simulink model "PubIfDecisionTOS_MDL"  (R2020b)
settings: configuration reference "DspaceConfig" (kept outside this file)
PostLoadFcn:
  | if any(exist('dsrtsu_mdlpostloadfcn', 'file') ~= 0), dsrtsu_mdlpostloadfcn('Execute', bdroot); end
InitFcn:
  | , if any(exist('dsmpb_private', 'file') ~= 0), dsmpb_private('dsmpb_mdlclblib', 'Init', bdroot); end,
undefined symbols (not defined in the file or in its folder): C_TOS_ACCEgoRAxletoFbumplength_m, C_TOS_ACCTargetFront_Flag, C_TOS_AEBJAPedObjDxThre_Val, C_TOS_AEBJAPedObjDyThre_Val, C_TOS_AEBJATargetSize_Val, C_TOS_AEBJAVehObjDxThre_Val, C_TOS_AEBJAVehObjDyThre_Val, C_TOS_AEBJuncPedTargetSize_Val, C_TOS_AEBLatObjDxThre_Val, C_TOS_AEBLatPedDyThre_Val, C_TOS_AEBLatTargetSize_Val, C_TOS_AEBLongTargetInEgoFront_Flag, C_TOS_axAbsGround_Parameter, C_TOS_CameraConfirmedFlag, C_TOS_CNsubjWidth, C_TOS_CurrentLaneCoreMinWidth_Val, C_TOS_CutInProb_Val_Zero, C_TOS_CutOutProb_Val_Zero, C_TOS_D2R_Val, C_TOS_DefaultValueObjectToCenterLine_dy, C_TOS_EgoCarWidth_Val, C_TOS_EgoDxRefPoint_m, C_TOS_EgoRAxletoFbumplength_m, C_TOS_HalfWidthVehicle_Con, C_TOS_HWA_CurrentLaneFlag, C_TOS_HWA_LeftLaneFlag, C_TOS_HWA_MovingDir_Vaild, C_TOS_HWA_MovState_Vaild, C_TOS_HWA_RightLaneFlag, C_TOS_LaneLineCourseErrorFront, C_TOS_LaneLineCourseErrorRear, C_TOS_MotorbikeDefaultWidth_m, C_TOS_NumberOfEffectiveTargets, C_TOS_Obj_Age_Val, C_TOS_Objdx_Constraint_Val, C_TOS_ObjectDefaultWidth_m, C_TOS_ObjInCurrentLane_Val, C_TOS_ObjInCurrentLaneValid, C_TOS_ObjInLeftLaneValid, C_TOS_ObjInRightLaneValid, C_TOS_ObjNotInCurrentLane_Val, C_TOS_ObjNotREElementType, C_TOS_ObjPredictDis_dy_ConstantVal_Zeros, C_TOS_ObjToCenterLine_ConstantVal_Zeros, C_TOS_OFMObjIDInvilad_Val, C_TOS_PIL_LatDisCons_Val_zero, C_TOS_PIL_ObjectCutInFlag_b, C_TOS_PIL_ObjectCutOutFlag_b, C_TOS_PIL_ObjLaneProb_al_Val, C_TOS_PP_ObjFusType_FC_Confirm_b, C_TOS_PP_ObjFusType_FC_FR_Confirm_b, C_TOS_PP_ObjFusType_FR_Confirm_b, C_TOS_RE_80BoolDefault_Val, C_TOS_RE_80Single181Default_Val, C_TOS_RE_80Single255Default_Val, C_TOS_RE_80Uint8Default_Val, C_TOS_RE_D2R, C_TOS_RE_D_180_Val, C_TOS_RE_InvalidObjectID_Val, C_TOS_RE_InvalidTargetChainDir_Val ... (+142)
libraries: simulink x1650, TOS_LIB x361, canfdmsglib x14
(part 66 of 69)

== stateflow chart PubIfDecisionTOS_MDL/TOS_20201112/TOS_2012080320/PP1128/AAT-AdditionalAttributes/RoadEdge/RE_2020_12_07/RoadEdge_V2/RoadEdgeGroupChain/EgoRight_RoadEdgeGroupChain ==
  state TargetChain_ObjDxDyAverageCal [function]
    state TCObjDxAve_Cal [function]
      (default) -> (junction 542) : {
          | j=uint8(1);
          | OFM_Object_Index = RE_StillObjectSortIndex[i] - uint8(1);
          | Start_Index_1 = OFM_Object_Index;
          | TargetChain_ObjectDx_1 = C_TOS_RE_80Single255Default_Val;
          | TargetChain_ObjectDx_2 = C_TOS_RE_80Single255Default_Val;
          | TargetChain_ObjectDx_3 = C_TOS_RE_80Single255Default_Val;
          | TargetChain_ObjectDx_4 = C_TOS_RE_80Single255Default_Val;
          | Sum_TargetChain_ObjectDx_1 = single(0);
          | Sum_TargetChain_ObjectDx_2 = single(0);
          | Sum_TargetChain_ObjectDx_3 = single(0);
          | Sum_TargetChain_ObjectDx_4 = single(0);
          | }
      (junction 542) -> (junction 543) [order 1] : [ j <= TargetChainElementNum[i] ]
      (junction 553) -> (junction 542) : {
          | j=j+uint8(1);
          | }
      (junction 542) -> (junction 552) [order 2]
      (junction 543) -> (junction 544) : {
          | StartDx_1 = ObjectDx[Start_Index_1];
          | TargetChain_ObjectDx_1[j] = ObjectDx[OFM_Object_Index];
          | }
      (junction 544) -> (junction 545) [order 1] : [TargetChain_ObjectDx_1[j] >= StartDx_1 &&...
          | abs(StartDx_1 - TargetChain_ObjectDx_1[j]) <= single(50)]
      (junction 544) -> (junction 546) [order 2] : {
          | Start_Index_2 = RE_StillObjectSortIndex[i+TargetChain_ObjectNum_1] - uint8(1);
          | StartDx_2 = ObjectDx[Start_Index_2];
          | TargetChain_ObjectDx_2[j] = ObjectDx[OFM_Object_Index];
          | }
      (junction 545) -> (junction 557) : {
          | TargetChainPart[i+j - uint8(1)] = uint8(1);
          | TargetChain_ObjectDx_1[j] = ObjectDx[OFM_Object_Index];
          | Sum_TargetChain_ObjectDx_1 = Sum_TargetChain_ObjectDx_1 + TargetChain_ObjectDx_1[j];
          | TargetChain_ObjectNum_1 = j;
          | OFM_Object_Index = RE_StillObjectSortIndex[i+j] - uint8(1);%索引值变到目标链上的下一个目标
          | }
      (junction 546) -> (junction 547) [order 1] : [TargetChain_ObjectDx_2[j] >= StartDx_2 &&...
          | abs(StartDx_2 - TargetChain_ObjectDx_2[j]) <= single(50)]
      (junction 546) -> (junction 548) [order 2] : {
          | Start_Index_3 = RE_StillObjectSortIndex[i + TargetChain_ObjectNum_1 + TargetChain_ObjectNum_2]  - uint8(1);
          | StartDx_3 = ObjectDx[Start_Index_3];
          | TargetChain_ObjectDx_3[j] = ObjectDx[OFM_Object_Index];
          | }
      (junction 547) -> (junction 556) : {
          | TargetChainPart[i+j - uint8(1)] = uint8(2);
          | TargetChain_ObjectDx_2[j] = ObjectDx[OFM_Object_Index];
          | Sum_TargetChain_ObjectDx_2 = Sum_TargetChain_ObjectDx_2 + TargetChain_ObjectDx_2[j];
          |  TargetChain_ObjectNum_2 = j - TargetChain_ObjectNum_1;
          | OFM_Object_Index = RE_StillObjectSortIndex[i+j] - uint8(1);%索引值变到目标链上的下一个目标
          | }
      (junction 548) -> (junction 549) [order 1] : [TargetChain_ObjectDx_3[j] >= StartDx_3 &&...
          | abs(StartDx_3 - TargetChain_ObjectDx_3[j]) <= single(50)]
      (junction 548) -> (junction 550) [order 2] : {
          | Start_Index_4 = RE_StillObjectSortIndex[i + TargetChain_ObjectNum_1 + TargetChain_ObjectNum_2 + TargetChain_ObjectNum_3]  - uint8(1);
          | StartDx_4 = ObjectDx[Start_Index_4];
          | TargetChain_ObjectDx_4[j] = ObjectDx[OFM_Object_Index];
          | }
      (junction 549) -> (junction 555) : {
          | TargetChainPart[i+j - uint8(1)] = uint8(3);
          | TargetChain_ObjectDx_3[j] = ObjectDx[OFM_Object_Index];
          | Sum_TargetChain_ObjectDx_3 = Sum_TargetChain_ObjectDx_3 + TargetChain_ObjectDx_3[j];
          |  TargetChain_ObjectNum_3 = j - TargetChain_ObjectNum_2 - TargetChain_ObjectNum_1 ;
          | OFM_Object_Index = RE_StillObjectSortIndex[i+j] - uint8(1);%索引值变到目标链上的下一个目标
          | }
      (junction 550) -> (junction 551) [order 1] : [TargetChain_ObjectDx_4[j] >= StartDx_4 &&...
          | abs(StartDx_4 - TargetChain_ObjectDx_4[j]) <= single(50)]
      (junction 550) -> (junction 553) [order 2] : {
          | TargetChainPart[i+j - uint8(1)]= uint8(0);
          | TargetChain_ObjectDx_Average_1 = single(255);
          | TargetChain_ObjectDx_Average_2 = single(255);
          | TargetChain_ObjectDx_Average_3 = single(255);
          | TargetChain_ObjectDx_Average_4 = single(255);
          | %同一目标链上的所有元素的Dx平均值，Dx平均值
          | }
      (junction 551) -> (junction 554) : {
          | TargetChainPart[i+j - uint8(1)]= uint8(4);
          | TargetChain_ObjectDx_4[j] = ObjectDx[OFM_Object_Index];
          | Sum_TargetChain_ObjectDx_4 = Sum_TargetChain_ObjectDx_4 + TargetChain_ObjectDx_4[j];
          | TargetChain_ObjectNum_4 = j - TargetChain_ObjectNum_3 - TargetChain_ObjectNum_2 - TargetChain_ObjectNum_1 ;
          | OFM_Object_Index = RE_StillObjectSortIndex[i+j] - uint8(1);%索引值变到目标链上的下一个目标
          | }
      (junction 554) -> (junction 553)
      (junction 555) -> (junction 554)
      (junction 556) -> (junction 555)
      (junction 557) -> (junction 556)
      (junction 552) -> (junction 558) : {
          | TargetChain_ObjectDx_Average_1 = Sum_TargetChain_ObjectDx_1/TargetChain_ObjectNum_1;
          | TargetChain_ObjectDx_Average_2 = Sum_TargetChain_ObjectDx_2/TargetChain_ObjectNum_2;
          | TargetChain_ObjectDx_Average_3 = Sum_TargetChain_ObjectDx_3/TargetChain_ObjectNum_3;
          | TargetChain_ObjectDx_Average_4 = Sum_TargetChain_ObjectDx_4/TargetChain_ObjectNum_4;
          | %同一目标链上的所有元素的Dx平均值，Dx平均值
          | }
    state TCObjDyAve_Cal [function]
      (default) -> (junction 481) : {
          | j=uint8(1);
          | OFM_Object_Index = RE_StillObjectSortIndex[i] - uint8(1);
          | Sum_TargetChain_ObjectDy = single(0);
          | }
      (junction 481) -> (junction 473) [order 1] : [ j <= TargetChainElementNum[i] ]
      (junction 475) -> (junction 481) : {
          | j=j+uint8(1);
          | }
      (junction 481) -> (junction 470) [order 2]
      (junction 473) -> (junction 475) : {
          | TargetChain_ObjectDy[j] = ObjectDy[OFM_Object_Index];
          | Sum_TargetChain_ObjectDy = Sum_TargetChain_ObjectDy + TargetChain_ObjectDy[j];
          | OFM_Object_Index = RE_StillObjectSortIndex[i+j] - uint8(1);
          | }
      (junction 470) -> (junction 480) : {
          | TargetChain_ObjectDy_Average[i] = Sum_TargetChain_ObjectDy/TargetChainElementNum[i];
          | %同一目标链上的所有元素的Dy平均值
          | }
    state TargetChain_ObjectDx_Average [function]
      state TargetChainPart4_DxAve [function]
        (default) -> (junction 626)
        (junction 626) -> (junction 635) [order 1] : [TargetChain_ObjectNum_4 <=uint8(2)]
        (junction 626) -> (junction 630) [order 2] : {
            | TargetChain_ObjectDx_Average[i] = TargetChain_ObjectDx_Average_4;
            | }
        (junction 635) -> (junction 633) : {
            | TargetChain_ObjectDx_Average[i] = (TargetChain_ObjectDx_Average_4+TargetChain_ObjectDx_Average_3)/2;
            | }
        (junction 633) -> (junction 630)
        (junction 630) -> (junction 636)
      state TargetChainPart3_DxAve [function]
        (default) -> (junction 655)
        (junction 655) -> (junction 653) [order 1] : [TargetChain_ObjectNum_3 <=uint8(2)]
        (junction 655) -> (junction 643) [order 2] : {
            | TargetChain_ObjectDx_Average[i] = TargetChain_ObjectDx_Average_3;
            | }
        (junction 653) -> (junction 644) : {
            | TargetChain_ObjectDx_Average[i] = (TargetChain_ObjectDx_Average_3+TargetChain_ObjectDx_Average_2)/2;
            | }
        (junction 644) -> (junction 643)
        (junction 643) -> (junction 645)
      state TargetChainPart2_DxAve [function]
        (default) -> (junction 672)
        (junction 672) -> (junction 674) [order 1] : [TargetChain_ObjectNum_2 <=uint8(2)]
        (junction 672) -> (junction 662) [order 2] : {
            | TargetChain_ObjectDx_Average[i] = TargetChain_ObjectDx_Average_2;
            | }
        (junction 674) -> (junction 663) : {
            | TargetChain_ObjectDx_Average[i] = (TargetChain_ObjectDx_Average_2+TargetChain_ObjectDx_Average_1)/2;
            | }
        (junction 663) -> (junction 662)
        (junction 662) -> (junction 664)
      (default) -> (junction 483)
      (junction 483) -> (junction 485) [order 1] : [TargetChainPart[i] == uint8(1)]
      (junction 483) -> (junction 491) [order 2]
      (junction 485) -> (junction 489) : {
          | TargetChain_ObjectDx_Average[i] = TargetChain_ObjectDx_Average_1;
          | }
      (junction 491) -> (junction 495) [order 1] : [TargetChainPart[i] == uint8(2)]
      (junction 491) -> (junction 493) [order 2]
      (junction 495) -> (junction 509) : {
          | TargetChainPart2_DxAve();
          | }
      (junction 493) -> (junction 497) [order 1] : [TargetChainPart[i] == uint8(3)]
      (junction 493) -> (junction 501) [order 2]
      (junction 497) -> (junction 499) : {
          | TargetChainPart3_DxAve();
          | }
      (junction 501) -> (junction 503) [order 1] : [TargetChainPart[i] == uint8(4)]
      (junction 501) -> (junction 487) [order 2] : {
          | TargetChain_ObjectDx_Average[i] = single(255);
          | }
      (junction 503) -> (junction 637) : {
          | TargetChainPart4_DxAve();
          | }
      (junction 637) -> (junction 487)
      (junction 499) -> (junction 637)
      (junction 509) -> (junction 499)
      (junction 489) -> (junction 509)
      (junction 487) -> (junction 513)
    (default) -> (junction 55)
    (junction 55) -> (junction 56) [order 1] : [ TargetChainStartIndex[i] != uint8(0)&&i == (TargetChainStartIndex[i]-uint8(1)) ]
        | %  i  目标 是目标链起始元素
    (junction 56) -> (junction 381) : {
        | TCObjDxAve_Cal();
        | TCObjDyAve_Cal();
        | }
    (junction 55) -> (junction 64) [order 2]
    (junction 64) -> (junction 66) [order 1] : [ (TargetChainStartIndex[i] != uint8(0))&&(i > (TargetChainStartIndex[i]-uint8(1)) )]
        | %目标i是目标链的剩余元素
    (junction 64) -> (junction 58) [order 2] : {
        | TargetChain_ObjectDx_Average[i] = single(255);
        | TargetChain_ObjectDy_Average[i] = single(255);
        | }
    (junction 66) -> (junction 68) : {
        | TargetChain_ObjectDx_Average();
        | TargetChain_ObjectDy_Average[i] = TargetChain_ObjectDy_Average[i - uint8(1)];
        | %同一目标链上的所有元素的Dx平均值，Dy平均值
        | }
    (junction 381) -> (junction 34) : {
        | TargetChain_ObjectDx_Average[i] = TargetChain_ObjectDx_Average_1;
        | }
    (junction 68) -> (junction 58)
    (junction 34) -> (junction 68)
    (junction 58) -> (junction 62)
  state RoadEdgeGroupChainJudge [function]
    (default) -> (junction 43) : {
        | OFM_Object_Index = RE_StillObjectSortIndex[i] - uint8(1);
        | }
    (junction 43) -> (junction 52) [order 1] : [abs(ObjectDx[OFM_Object_Index] - TargetChain_ObjectDx_Average[i]) < P_TOS_RE_RoadEdgeGroupDxThre_Val]
    (junction 43) -> (junction 47) [order 2] : {
        | REGroupChainFlag[i] =false;
        | }
    (junction 52) -> (junction 74)
    (junction 74) -> (junction 76) [order 1] : [Ego_Velocity > P_TOS_RE_RoadEdgeGroupEgoVxvThre_Val&&...
        | (abs(ObjectDy[OFM_Object_Index] - TargetChain_ObjectDy_Average[i]) < P_TOS_RE_RoadEdgeGroupDy_HighSpeedThre_Val)]
    (junction 74) -> (junction 78) [order 2]
    (junction 76) -> (junction 84) : {
        | REGroupChainFlag[i] = true;
        | }
    (junction 78) -> (junction 80) [order 1] : [Ego_Velocity <= P_TOS_RE_RoadEdgeGroupEgoVxvThre_Val &&...
        | (abs(ObjectDy[OFM_Object_Index] - TargetChain_ObjectDy_Average[i]) < P_TOS_RE_RoadEdgeGroupDy_LowSpeedThre_Val)]
    (junction 78) -> (junction 86) [order 2] : {
        | REGroupChainFlag[i] =false;
        | }
    (junction 80) -> (junction 82) : {
        | REGroupChainFlag[i] = true;
        | }
    (junction 86) -> (junction 47)
    (junction 82) -> (junction 86)
    (junction 84) -> (junction 82)
    (junction 47) -> (junction 93)
  state REGroupChainNumCal [function]
    note: 计算连续满足条件的边界组链的元素个数
        | 给边界组链中元素编号
    note: 3个目标组成一条链目标连；
        | 计算得到目标链的起始目标在Dx排序中的Index+1；
    (default) -> (junction 204)
    (junction 204) -> (junction 205) [order 1] : [i == uint8(0)]
        | %从每个目标链的第一个元素开始计数
    (junction 204) -> (junction 581) [order 2]
    (junction 205) -> (junction 211)
    (junction 581) -> (junction 584) [order 1] : [i > uint8(0)&&...
        | TargetChainStartIndex[i] !=uint8(0)&&...
        | TargetChainStartIndex[i-uint8(1)] !=uint8(0)&&...
        | TargetChainStartIndex[i] != TargetChainStartIndex[i - uint8(1)]]
        | %从每个目标链的第一个元素开始计数
    (junction 581) -> (junction 122) [order 2]
    (junction 584) -> (junction 589)
    (junction 589) -> (junction 598) [order 1] : [REGroupChainFlag[i] == true]
    (junction 211) -> (junction 213) [order 1] : [REGroupChainFlag[i] == true]
    (junction 122) -> (junction 123) [order 1] : [REGroupChainFlag[i] == true]
    (junction 589) -> (junction 597) [order 2] : {
        | GroupChainElementCounter[i] = uint8(0);
        | }
    (junction 598) -> (junction 594) : {
        | GroupChainElementCounter[i] = uint8(1);
        | }
    (junction 211) -> (junction 208) [order 2] : {
        | GroupChainElementCounter[i] = uint8(0);
        | }
    (junction 213) -> (junction 215) : {
        | GroupChainElementCounter[i] = uint8(1);
        | }
    (junction 122) -> (junction 124) [order 2] : {
        | GroupChainElementCounter[i] = uint8(0);
        | }
    (junction 123) -> (junction 125) : {
        | GroupChainElementCounter[i] = GroupChainElementCounter[i-uint8(1)] + uint8(1);
        | }
    (junction 125) -> (junction 124)
    (junction 597) -> (junction 125)
    (junction 594) -> (junction 597)
    (junction 208) -> (junction 594)
    (junction 215) -> (junction 208)
    (junction 124) -> (junction 126)
    (junction 126) -> (junction 127) [order 1] : [GroupChainElementCounter[i] == uint8(3)]
        | %连续3个目标符合条件时，组成边界组链；
    (junction 126) -> (junction 128) [order 2]
    (junction 127) -> (junction 132) : {
        | GroupChainStartIndex[i - uint8(2)] = i - uint8(1);
        | GroupChainStartIndex[i - uint8(1)] = i - uint8(1);
        | GroupChainStartIndex[i] = i - uint8(1) ;
        | %GroupChainElementCounter[i - uint8(2)] = uint8(1);
        | %GroupChainElementCounter[i - uint8(1)] = uint8(2);
        | %边界组链元素起始目标Index从1开始计数
        | }
    (junction 128) -> (junction 129) [order 1] : [GroupChainElementCounter[i]  > uint8(3)]
    (junction 128) -> (junction 130) [order 2] : {
        | GroupChainStartIndex[i] = uint8(0);
        | %GroupChainElementCounter[i] = uint8(0);
        | }
    (junction 129) -> (junction 131) : {
        | GroupChainStartIndex[i] = GroupChainStartIndex[i - uint8(1)] ;
        | %边界组链元素i序号不变
        | }
    (junction 131) -> (junction 130)
    (junction 132) -> (junction 131)
    (junction 130) -> (junction 226)
  (default) -> (junction 2) : {
      | i = uint8(0);
      | TargetChainPart = C_TOS_RE_80Uint8Default_Val;
      | TargetChain_ObjectDx_Average = C_TOS_RE_80Single255Default_Val;
      | TargetChain_ObjectDy_Average = C_TOS_RE_80Single255Default_Val;
      | REGroupChainFlag = C_TOS_RE_80BoolDefault_Val;
      | GroupChainElementCounter = C_TOS_RE_80Uint8Default_Val;
      | GroupChainStartIndex = C_TOS_RE_80Uint8Default_Val;
      | }
      | %从第1个目标开始
  (junction 2) -> (junction 3) [order 1] : [RE_StillObjectSortIndex[i] ~= C_TOS_StillObjSortInvalidIndex_Val&&...
      | i <= uint8(79)]
  (junction 118) -> (junction 2) : {
      | i = i+uint8(1);
      | }
  (junction 2) -> (junction 5) [order 2]
  (junction 3) -> (junction 38) : {
      | TargetChain_ObjDxDyAverageCal();
      | }
  (junction 38) -> (junction 7) : {
      | RoadEdgeGroupChainJudge();
      | }
  (junction 7) -> (junction 118) : {
      | REGroupChainNumCal();
      | }
  (junction 5) -> (junction 10)
  data: GroupChainElementCounter output uint8 size=80; GroupChainStartIndex output uint8 size=80; C_TOS_StillObjSortInvalidIndex_Val parameter; ObjectDx input size=80; ObjectDy input size=80; P_TOS_RE_RoadEdgeGroupDxThre_Val parameter; RE_StillObjectSortIndex input size=80; TargetChainElementNum input size=80; TargetChainStartIndex input size=80; REGroupChainFlag output uint8 size=80; OFM_Object_Index local uint8 size=1; TargetChain_ObjectDy local single size=80; i local uint8 size=1; j local uint8 size=1; Ego_Velocity input size=1; P_TOS_RE_RoadEdgeGroupDy_HighSpeedThre_Val parameter; P_TOS_RE_RoadEdgeGroupDy_LowSpeedThre_Val parameter; P_TOS_RE_RoadEdgeGroupEgoVxvThre_Val parameter; Sum_TargetChain_ObjectDy local single size=1; RE_TargetChainIndex input uint8 size=80; C_TOS_RE_80Single255Default_Val parameter; C_TOS_RE_80BoolDefault_Val parameter; C_TOS_RE_80Uint8Default_Val parameter; StartDx_1 local single size=1 =255; StartDx_2 local single size=1 =255; StartDx_3 local single size=1 =255; StartDx_4 local single size=1 =255; Start_Index_1 local uint8 size=1 =0; Start_Index_2 local uint8 size=1 =0; Start_Index_3 local uint8 size=1 =0; Start_Index_4 local uint8 size=1 =0; Sum_TargetChain_ObjectDx_1 local single size=1 =0; Sum_TargetChain_ObjectDx_2 local single size=1 =0; Sum_TargetChain_ObjectDx_3 local single size=1 =0; Sum_TargetChain_ObjectDx_4 local single size=1 =0; TargetChain_ObjectDx_1 local single size=80 =255; TargetChain_ObjectDx_2 local single size=80 =255; TargetChain_ObjectDx_3 local single size=80 =255; TargetChain_ObjectDx_4 local single size=80 =255; TargetChain_ObjectDx_Average_1 local single size=1 =255; TargetChain_ObjectDx_Average_2 local single size=1 =255; TargetChain_ObjectDx_Average_3 local single size=1 =255; TargetChain_ObjectDx_Average_4 local single size=1 =255; TargetChain_ObjectNum_1 local uint8 size=1 =0; TargetChain_ObjectNum_2 local uint8 size=1 =0; TargetChain_ObjectNum_3 local uint8 size=1 =0; TargetChain_ObjectNum_4 local uint8 size=1 =0; TargetChain_ObjectDx_Average output single size=80; TargetChain_ObjectDy_Average output single size=80; TargetChainPart output uint8 size=80 =0

== stateflow chart PubIfDecisionTOS_MDL/TOS_20201112/TOS_2012080320/PP1128/AAT-AdditionalAttributes/RoadEdge/RE_2020_12_07/RoadEdge_V2/RoadEdgeGroupChain/EgoRight_RoadEdgeGroupChainInfo ==
  state REGroupChainNumCal [function]
    note: 给边界组链编号
    (default) -> (junction 181)
    (junction 181) -> (junction 190) [order 1] : [i == uint8(0)]
        | %Dx最近的目标是边界组链开始元素
    (junction 181) -> (junction 133) [order 2]
    (junction 190) -> (junction 195)
    (junction 195) -> (junction 185) [order 1] : [GroupChainStartIndex[i] != uint8(0)]
    (junction 195) -> (junction 192) [order 2] : {
        | GroupChainIndex[i] = uint8(0);
        | }
    (junction 185) -> (junction 188) : {
        | GroupChainIndex[i] = GroupChainNum;
        |  GroupChainNum = GroupChainNum + uint8(1);
        | }
    (junction 133) -> (junction 134) [order 1] : [(GroupChainStartIndex[i-uint8(1)] == uint8(0)&&...
        | GroupChainStartIndex[i] != uint8(0))||...
        | (GroupChainStartIndex[i-uint8(1)] != uint8(0)&&...
        | GroupChainStartIndex[i] != uint8(0)&&...
        | GroupChainStartIndex[i] != GroupChainStartIndex[i-uint8(1)])]
        | %边界组链开始元素
    (junction 133) -> (junction 135) [order 2]
    (junction 134) -> (junction 139) : {
        | GroupChainIndex[i] = GroupChainNum;
        |  GroupChainNum = GroupChainNum + uint8(1);
        | }
    (junction 135) -> (junction 136) [order 1] : [GroupChainStartIndex[i] != uint8(0)&&...
        | GroupChainStartIndex[i] == GroupChainStartIndex[i-uint8(1)]]
        | %边界组链剩余元素
    (junction 135) -> (junction 137) [order 2] : {
        | GroupChainIndex[i] = uint8(0);
        | }
    (junction 136) -> (junction 138) : {
        | GroupChainIndex[i] = GroupChainIndex[i-uint8(1)];
        | }
    (junction 138) -> (junction 137)
    (junction 139) -> (junction 138)
    (junction 192) -> (junction 139)
    (junction 188) -> (junction 192)
    (junction 137) -> (junction 140)
  state REGroupChainElementNumCal [function]
    (default) -> (junction 198)
    (junction 198) -> (junction 197) [order 1] : [i > uint8(1)]
    (junction 198) -> (junction 201) [order 2] : {
        | GroupChainElementNum[i] = uint8(0);
        | }
    (junction 197) -> (junction 169)
    (junction 169) -> (junction 170) [order 1] : [(GroupChainStartIndex[i-uint8(1)] != uint8(0)&&...
        | GroupChainStartIndex[i] == uint8(0))||...
        | (GroupChainStartIndex[i-uint8(1)] != uint8(0)&&...
        | GroupChainStartIndex[i] != GroupChainStartIndex[i-uint8(1)])]
        | %[i-uint8(1)]为目标链结束元素
    (junction 169) -> (junction 171) [order 2] : {
        | GroupChainElementNum[i-uint8(1)] = uint8(0);
        | }
    (junction 170) -> (junction 172) : {
        | GroupChainElementNum[i-uint8(1)] = GroupChainElementCounter[i-uint8(1)] ;
        | }
    (junction 171) -> (junction 201)
    (junction 172) -> (junction 171)
    (junction 201) -> (junction 173)
    (junction 173) -> (junction 237) [order 1] : [i > uint8(2)&&GroupChainElementNum[i-uint8(1)]  != uint8(0)]
        | %边界组链结束元素，从第3个目标开始判断，[i]目标为边界组链结束元素
    (junction 173) -> (junction 240) [order 2]
    (junction 237) -> (junction 239) : {
        | j = uint8(1);
        | }
    (junction 239) -> (junction 235) [order 1] : [ j <= GroupChainElementNum[i-uint8(1)] ]
    (junction 231) -> (junction 239) : {
        | j = j+uint8(1);
        | }
    (junction 239) -> (junction 233) [order 2]
    (junction 235) -> (junction 231) : {
        | GroupChainElementNum[i-j] = GroupChainElementNum[i-uint8(1)];
        | }
        | %同一目标链上所有元素标记目标链的元素个数
    (junction 233) -> (junction 240)
    (junction 240) -> (junction 242)
  (default) -> (junction 2) : {
      | i = uint8(0);
      | GroupChainNum=uint8(1);
      | GroupChainIndex = C_TOS_RE_80Uint8Default_Val;
      | GroupChainElementNum = C_TOS_RE_80Uint8Default_Val;
      | }
      | %从第1个目标开始
  (junction 2) -> (junction 3) [order 1] : [(RE_StillObjectSortIndex[i] ~= C_TOS_StillObjSortInvalidIndex_Val||...
      | (i > uint8(0)&&RE_StillObjectSortIndex[i-uint8(1)] ~= C_TOS_StillObjSortInvalidIndex_Val))&&...
      | i <= uint8(79)]
      | %循环到有效目标的下一个目标，保证找到边界组链的结束元素
  (junction 116) -> (junction 2) : {
      | i = i+uint8(1);
      | }
  (junction 2) -> (junction 5) [order 2]
  (junction 3) -> (junction 118) : {
      | REGroupChainNumCal();
      | }
  (junction 118) -> (junction 116) : {
      | REGroupChainElementNumCal();
      | }
  (junction 5) -> (junction 10)
  data: GroupChainIndex output uint8 size=80; C_TOS_StillObjSortInvalidIndex_Val parameter; RE_StillObjectSortIndex input size=80; i local uint8 size=1; GroupChainElementCounter input uint8 size=80; GroupChainStartIndex input uint8 size=80; GroupChainElementNum output uint8 size=80; GroupChainNum local uint8 size=1; C_TOS_RE_80Uint8Default_Val parameter; j local uint8 size=1

== matlab function PubIfDecisionTOS_MDL/TOS_20201112/TOS_2012080320/PP1128/AAT-AdditionalAttributes/RoadEdge/RE_2020_12_07/RoadEdge_V2/SelectStationaryObjects/MATLAB Function3 ==
  data: Object_Num input; ObjectCondFlag input; Object_Dx input; ObjDisIndex_Left output; Object_Dy input; ObjDisIndex_Right output
function [ObjDisIndex_Left ,ObjDisIndex_Right] = fcn(Object_Num,ObjectCondFlag,Object_Dx,Object_Dy)
ObjNum=80;
ObjDisIndex_Left=uint8(zeros(ObjNum,1));
Dx_Left=Object_Dx;
MidIndex_Left=1:1:ObjNum;

ObjDisIndex_Right=uint8(zeros(ObjNum,1));
Dx_Right=Object_Dx;
MidIndex_Right=1:1:ObjNum;

            if ObjectCondFlag(Object_Num) == false || Object_Dy(Object_Num) < single(-0.5)
                 Dx_Left(Object_Num) = single(255);
            end
            if ObjectCondFlag(Object_Num) == false || Object_Dy(Object_Num) > single(0.5)
                Dx_Right(Object_Num) = single(255);
            end
for i=1:Object_Num
    %% 对所有不符合排序条件的目标Dx值255
    
    if ObjectCondFlag(i) == false || Object_Dy(i) < single(-0.5)
        Dx_Left(i) = single(255);
    end
    if ObjectCondFlag(i) == false || Object_Dy(i) > single(0.5)
        Dx_Right(i) = single(255);
    end

    %% 
    
    
    ObjDisIndex_Left(i)=MidIndex_Left(i);
    t_dis_left=Dx_Left(i);
    
    ObjDisIndex_Right(i)=MidIndex_Right(i);
    t_dis_Right=Dx_Right(i);
    
    if i<Object_Num-1
        for j=(i+1):Object_Num
            
                if ObjectCondFlag(j) == false||Object_Dy(j) < (single(-0.5))
                    Dx_Left(j) = single(255);
                end
                if ObjectCondFlag(j) == false || Object_Dy(j) > (single(0.5))
                   Dx_Right(j) = single(255);
                end

            if Dx_Left(j)<t_dis_left
                temp_index_Left=ObjDisIndex_Left(i);
                temp_dis_Left=t_dis_left;
                
                ObjDisIndex_Left(i)=MidIndex_Left(j);
                Dx_Left(i)=Dx_Left(j);
                t_dis_left=Dx_Left(j);
                MidIndex_Left(j)=temp_index_Left;
                Dx_Left(j)=temp_dis_Left;
            end
            
            if Dx_Right(j)<t_dis_Right
                temp_index_Right=ObjDisIndex_Right(i);
                temp_dis_Right=t_dis_Right;
                ObjDisIndex_Right(i)=MidIndex_Right(j);
                Dx_Right(i)=Dx_Right(j);
                t_dis_Right=Dx_Right(j);
                MidIndex_Right(j)=temp_index_Right;
                Dx_Right(j)=temp_dis_Right;
            end
            
            if Dx_Left(i) >= single(250)     
                ObjDisIndex_Left(i)=uint8(0); 
            end   
            if Dx_Right(i) >= single(250)     
                ObjDisIndex_Right(i)=uint8(0); 
            end   
   
        end
    else
           
            
        if i~=Object_Num
            if Dx_Left(Object_Num)<t_dis_left
                temp_index_Left=ObjDisIndex_Left(i);
                temp_dis_Left=t_dis_left;
                ObjDisIndex_Left(i)=MidIndex_Left(Object_Num);
                Dx_Left(i)=Dx_Left(Object_Num);
                MidIndex_Left(Object_Num)=temp_index_Left;
                Dx_Left(Object_Num)=temp_dis_Left;
            else
                MidIndex_Left(Object_Num)=MidIndex_Left(Object_Num);
                Dx_Left(Object_Num)=Dx_Left(Object_Num);
            end
            
            if Dx_Left(i) >= single(250)     
                ObjDisIndex_Left(i)=uint8(0); 
            end   
            
            
            if Dx_Right(Object_Num)<t_dis_Right
                temp_index_Right=ObjDisIndex_Right(i);
                temp_dis_Right=t_dis_Right;
                ObjDisIndex_Right(i)=MidIndex_Right(Object_Num);
                Dx_Right(i)=Dx_Right(Object_Num);
                MidIndex_Right(Object_Num)=temp_index_Right;
                Dx_Right(Object_Num)=temp_dis_Right;
            else
                MidIndex_Right(Object_Num)=MidIndex_Right(Object_Num);
                Dx_Right(Object_Num)=Dx_Right(Object_Num);
            end
            
            if Dx_Right(i) >= single(250)     
                ObjDisIndex_Right(i)=uint8(0); 
            end    

        end
    end
            
end
if Dx_Right(Object_Num) >= single(250)     
    ObjDisIndex_Right(Object_Num)=uint8(0); 
end   
if Dx_Left(Object_Num) >= single(250)     
   ObjDisIndex_Left(Object_Num)=uint8(0); 
end

== stateflow chart PubIfDecisionTOS_MDL/TOS_20201112/TOS_2012080320/PP1128/AAT-AdditionalAttributes/RoadEdge/RE_2020_12_07/RoadEdge_V2/SelectStationaryObjects/SelectStationaryObject/RE_StationaryObjectsSortCond/Subsystem/StateDelayAbortion ==
  state NormalState
    en:
    stateOut = state;
    CNTimeCounterMAX = 256;
    du:
    stateOut = state;
  state CounterState
    en:
    timeSinceLastState = 0;
    state_K1 = stateK1;
    du:
    timeSinceLastState +=  Ts;
    CounterStateFunc();
  state CounterStateFunc [function]
    (default) -> (junction 70)
    (junction 70) -> (junction 62) [order 1] : [timeSinceLastState > CNTimeCounterMAX]
    (junction 70) -> (junction 69) [order 2] : %do nothing
    (junction 62) -> (junction 61) : {
        | 	timeSinceLastState = CNTimeCounterMAX;
        | }
    (junction 61) -> (junction 69)
    (junction 69) -> (junction 68)
    (junction 68) -> (junction 60) [order 1] : [timeSinceLastState <= stateProlongationTime]
    (junction 68) -> (junction 66) [order 2] : {
        | 	stateOut = state;
        | }
    (junction 60) -> (junction 67) : {
        | 	stateOut = state_K1;
        | }
    (junction 67) -> (junction 66)
    (junction 66) -> (junction 56)
  (default) -> NormalState
  NormalState -> CounterState : [stateK1 != uint8(0) &&...
      | state == uint8(0)]
  CounterState -> NormalState : [timeSinceLastState > stateProlongationTime]
  data: state input; stateK1 input; stateProlongationTime input; timeSinceLastState output double; stateOut output uint8; Ts input; CNTimeCounterMAX local double; state_K1 local uint8

== stateflow chart PubIfDecisionTOS_MDL/TOS_20201112/TOS_2012080320/PP1128/AAT-AdditionalAttributes/RoadEdge/RE_2020_12_07/RoadEdge_V2/TargetChain/EgoLeftTargetChainDirection/TargetChainDirectionCalCulat ==
  note: RE_TargetChainDir
      | 0:Invalid
      | 1:Stright_Same  Dir
      | 2:Stright_Different Dir
      | 3:Left_Same  Dir
      | 4:Left_Different Dir
      | 5:Right_Same  Dir
      | 6:Right_Different Dir
  note: RE_TargetChainStartDir:
      |
      | 0:Invalid
      | 1:Stright Dir
      | 2:Left Dir
      | 3:Right Dir
  state TargetChainStartDirJudge [function]
    note: RE_TargetChainStartDir:
        |
        | 0:Invalid
        | 1:Stright  Dir
        | 2:Left Dir
        | 3:Right Dir
    (default) -> (junction 76)
    (junction 76) -> (junction 75) [order 1] : [RE_StillTarget_Theta2_ALL[i] < P_TOS_RE_StrightDirThetaMax_val &&...
        | RE_StillTarget_Theta2_ALL[i] > P_TOS_RE_StrightDirThetaMin_val]
    (junction 75) -> (junction 63) : {
        | RE_TargetChainStartDir[i] = uint8(1);
        | }
    (junction 76) -> (junction 68) [order 2]
    (junction 68) -> (junction 77) [order 1] : [RE_StillTarget_Theta2_ALL[i] <= P_TOS_RE_StrightDirThetaMin_val&&...
        | RE_StillTarget_Theta2_ALL[i] > single(-1)*C_TOS_RE_ThretaDefault_Val]
    (junction 68) -> (junction 64) [order 2]
    (junction 77) -> (junction 62) : {
        | RE_TargetChainStartDir[i]  = uint8(2);
        | }
    (junction 64) -> (junction 58) [order 1] : [RE_StillTarget_Theta2_ALL[i] >= P_TOS_RE_StrightDirThetaMax_val &&...
        | RE_StillTarget_Theta2_ALL[i] < C_TOS_RE_ThretaDefault_Val]
    (junction 64) -> (junction 59) [order 2] : {
        | RE_TargetChainStartDir[i]  = uint8(0);
        | }
        | %donothing
    (junction 58) -> (junction 61) : {
        | RE_TargetChainStartDir[i]  = uint8(3);
        | }
    (junction 63) -> (junction 62)
    (junction 61) -> (junction 59)
    (junction 62) -> (junction 61)
    (junction 59) -> (junction 80)
  state Target2ChainDirJudge [function]
    note: RE_TargetChainDir
        | 0:Invalid
        | 1:Stright_Same  Dir
        | 2:Stright_Different Dir
        | 3:Left_Same  Dir
        | 4:Left_Different Dir
        | 5:Right_Same  Dir
        | 6:Right_Different Dir
    state RightDir_TargetDirJudge [function]
      (default) -> (junction 282)
      (junction 282) -> (junction 285) [order 1] : [RE_StillTarget_Theta2_ALL[i] < P_TOS_RE_StrightDirThetaMax_val &&...
          | RE_StillTarget_Theta2_ALL[i] > P_TOS_RE_StrightDirThetaMin_val]
      (junction 282) -> (junction 300) [order 2]
      (junction 285) -> (junction 299) : {
          | RE_TargetChainDir[i] = uint8(5);
          | }
      (junction 300) -> (junction 286) [order 1] : [RE_StillTarget_Theta2_ALL[i] <= P_TOS_RE_StrightDirThetaMin_val &&...
          | RE_StillTarget_Theta2_ALL[i] > single(-1)*C_TOS_RE_ThretaDefault_Val]
      (junction 300) -> (junction 297) [order 2]
      (junction 286) -> (junction 289) : {
          | RE_TargetChainDir[i] = uint8(6);
          | }
      (junction 297) -> (junction 295) [order 1] : [RE_StillTarget_Theta2_ALL[i] >= P_TOS_RE_StrightDirThetaMax_val &&...
          | RE_StillTarget_Theta2_ALL[i]< C_TOS_RE_ThretaDefault_Val]
      (junction 297) -> (junction 278) [order 2] : {
          | RE_TargetChainDir[i] = uint8(0);
          | }%donothing
      (junction 295) -> (junction 292) : {
          | RE_TargetChainDir[i] = uint8(6);
          | }
      (junction 292) -> (junction 278)
      (junction 289) -> (junction 292)
      (junction 299) -> (junction 289)
      (junction 278) -> (junction 223)
    state LeftDir_TargetDirJudge [function]
      (default) -> (junction 256)
      (junction 256) -> (junction 258) [order 1] : [RE_StillTarget_Theta2_ALL[i] < P_TOS_RE_StrightDirThetaMax_val &&...
          | RE_StillTarget_Theta2_ALL[i] > P_TOS_RE_StrightDirThetaMin_val]
      (junction 256) -> (junction 265) [order 2]
      (junction 258) -> (junction 259) : {
          | RE_TargetChainDir[i] = uint8(3);
          | }
      (junction 265) -> (junction 267) [order 1] : [RE_StillTarget_Theta2_ALL[i] <= P_TOS_RE_StrightDirThetaMin_val &&...
          | RE_StillTarget_Theta2_ALL[i] > single(-1)*C_TOS_RE_ThretaDefault_Val]
      (junction 265) -> (junction 261) [order 2]
      (junction 267) -> (junction 273) : {
          | RE_TargetChainDir[i]  = uint8(4);
          | }
      (junction 261) -> (junction 270) [order 1] : [RE_StillTarget_Theta2_ALL[i] >= P_TOS_RE_StrightDirThetaMax_val &&...
          | RE_StillTarget_Theta2_ALL[i ]< C_TOS_RE_ThretaDefault_Val]
      (junction 261) -> (junction 254) [order 2] : {
          | RE_TargetChainDir[i] = uint8(0);
          | }%donothing
      (junction 270) -> (junction 268) : {
          | RE_TargetChainDir[i]  = uint8(4);
          | }
      (junction 259) -> (junction 273)
      (junction 273) -> (junction 268)
      (junction 268) -> (junction 254)
      (junction 254) -> (junction 276)
    state StrightDir_TargetDirJudge [function]
      (default) -> (junction 233)
      (junction 233) -> (junction 235) [order 1] : [RE_StillTarget_Theta2_ALL[i] < P_TOS_RE_StrightDirThetaMax_val &&...
          | RE_StillTarget_Theta2_ALL[i] > P_TOS_RE_StrightDirThetaMin_val]
      (junction 233) -> (junction 239) [order 2]
      (junction 235) -> (junction 230) : {
          | RE_TargetChainDir[i] = uint8(1);
          | }
      (junction 239) -> (junction 238) [order 1] : [RE_StillTarget_Theta2_ALL[i] <= P_TOS_RE_StrightDirThetaMin_val &&...
          | RE_StillTarget_Theta2_ALL[i] > single(-1)*C_TOS_RE_ThretaDefault_Val]
      (junction 239) -> (junction 243) [order 2]
      (junction 238) -> (junction 241) : {
          | RE_TargetChainDir[i] = uint8(2);
          | }
      (junction 243) -> (junction 227) [order 1] : [RE_StillTarget_Theta2_ALL[i] >= P_TOS_RE_StrightDirThetaMax_val &&...
          | RE_StillTarget_Theta2_ALL[i ]< C_TOS_RE_ThretaDefault_Val]
      (junction 243) -> (junction 229) [order 2] : {
          | RE_TargetChainDir[i] = uint8(0);
          | }%donothing
      (junction 227) -> (junction 246) : {
          | RE_TargetChainDir[i] = uint8(2);
          | }
      (junction 246) -> (junction 229)
      (junction 241) -> (junction 246)
      (junction 230) -> (junction 241)
      (junction 229) -> (junction 249)
    (default) -> (junction 114)
    (junction 114) -> (junction 113) [order 1] : [RE_TargetChainStartDir[i-uint8(1)] == uint8(1)]
    (junction 114) -> (junction 115) [order 2]
    (junction 113) -> (junction 250) : {
        | StrightDir_TargetDirJudge();
        | }
    (junction 115) -> (junction 116) [order 1] : [RE_TargetChainStartDir[i-uint8(1)]  == uint8(2)]
    (junction 115) -> (junction 117) [order 2]
    (junction 116) -> (junction 302) : {
        | LeftDir_TargetDirJudge();
        | }
    (junction 117) -> (junction 118) [order 1] : [RE_TargetChainStartDir[i-uint8(1)]  == uint8(3)]
    (junction 117) -> (junction 120) [order 2] : {
        | RE_TargetChainDir[i] = uint8(0);
        | }%donothing
    (junction 118) -> (junction 304) : {
        | RightDir_TargetDirJudge();
        | }
    (junction 304) -> (junction 120)
    (junction 302) -> (junction 304)
    (junction 250) -> (junction 302)
    (junction 120) -> (junction 123)
  (default) -> (junction 41)
  (junction 41) -> (junction 42) : {
      | i=uint8(1);
      | RE_TargetChainStartDir = C_TOS_RE_80Uint8Default_Val;
      | RE_TargetChainDir = C_TOS_RE_80Uint8Default_Val;
      |  }
      | %从第2个目标开始判断目标链起始方向
  (junction 42) -> (junction 47) [order 1] : [RE_StationaryObjectsSortIndex[i] ~= C_TOS_StillObjSortInvalidIndex_Val &&...
      | i <= uint8(79)]
  (junction 50) -> (junction 42) : {
      | i=i+uint8(1);
      | }
  (junction 42) -> (junction 44) [order 2]
  (junction 47) -> (junction 330) : {
      | TargetChainStartDirJudge();
      | }
  (junction 330) -> (junction 332) [order 1] : [i > uint8(1)]
      | %从第3个目标开始,判断目标链方向
  (junction 330) -> (junction 50) [order 2] : {
      | RE_TargetChainDir[i] = uint8(0);
      | }
  (junction 332) -> (junction 333) : {
      | Target2ChainDirJudge();
      | }
  (junction 333) -> (junction 50)
  (junction 44) -> (junction 45)
  data: RE_StationaryObjectsSortIndex input uint8 size=80; P_TOS_RE_StrightDirThetaMax_val parameter; C_TOS_RE_ThretaDefault_Val parameter; P_TOS_RE_StrightDirThetaMin_val parameter; RE_TargetChainStartDir output uint8 size=80; RE_TargetChainDir output uint8 size=80; i local uint8 size=1; RE_StillTarget_Theta2_ALL input single size=80; C_TOS_StillObjSortInvalidIndex_Val parameter; C_TOS_RE_80Uint8Default_Val parameter

== stateflow chart PubIfDecisionTOS_MDL/TOS_20201112/TOS_2012080320/PP1128/AAT-AdditionalAttributes/RoadEdge/RE_2020_12_07/RoadEdge_V2/TargetChain/EgoLeftTargetChainDirection/Theta_Calculation ==
  state StillTarget12_0_Theta = Theta_Cal(ObjectsSortIndex,ObjectsSortIndex_K1,StillTarget2_Dx,StillTarget1_Dx,StillTarget2_Dy,StillTarget1_Dy,RE_2TargetTheta_K1) [function]
  (default) -> (junction 2) : {
      | i=uint8(1);
      | StillTarget12_0_Theta_ALL = C_TOS_RE_80Single181Default_Val;
      | StillTarget12_0_Theta_ALL[0] = single(90);
      | StillTarget23_12_Theta_ALL = C_TOS_RE_80Single181Default_Val;
      | }
      | %从第2个目标开始   1
  (junction 2) -> (junction 3) [order 1] : [RE_StationaryObjectsSortIndex[i] ~= C_TOS_StillObjSortInvalidIndex_Val &&...
      | i <= uint8(79)]
  (junction 76) -> (junction 2) : {
      | i = i+uint8(1);
      | }
  (junction 2) -> (junction 7) [order 2]
  (junction 3) -> (junction 33) : {
      | StillTarget1_Index=RE_StationaryObjectsSortIndex[i-uint8(1)];
      | StillTarget2_Index=RE_StationaryObjectsSortIndex[i];
      | }
  (junction 33) -> (junction 12) : {
      | StillTarget1_Dx = Object_Dx[StillTarget1_Index-uint8(1)];
      | StillTarget2_Dx = Object_Dx[StillTarget2_Index-uint8(1)];
      | StillTarget1_Dy = Object_Dy[StillTarget1_Index-uint8(1)];
      | StillTarget2_Dy = Object_Dy[StillTarget2_Index-uint8(1)];
      | }
      | %提取相邻两个点的Dx，Dy
  (junction 12) -> (junction 74) : {
      | ObjectsSortIndex_K1 = RE_StationaryObjectsSortIndex_K1[i];
      | ObjectsSortIndex = RE_StationaryObjectsSortIndex[i];
      | RE_2TargetTheta_K1 = RE_2TargetTheta_ALL_K1[i];
      | StillTarget12_0_Theta = Theta_Cal(ObjectsSortIndex,ObjectsSortIndex_K1,StillTarget2_Dx,StillTarget1_Dx,StillTarget2_Dy,StillTarget1_Dy,RE_2TargetTheta_K1);
      | StillTarget12_0_Theta_ALL[i] = StillTarget12_0_Theta;
      | }
      | %计算相邻两个点的直线与dy轴夹角，角度范围，顺时针0-180度
  (junction 74) -> (junction 76) : {
      | StillTarget23_12_Theta = StillTarget12_0_Theta_ALL[i] - StillTarget12_0_Theta_ALL[i-uint8(1)];
      | StillTarget23_12_Theta_ALL[i] = StillTarget23_12_Theta;
      | }
      | %计算2，3点连线的斜率角减去第1，2点连线之间的斜率角，角度范围+-180度
      | %StillTarget23_12_Theta_ALL元素对应按Dx从小到大的顺序排列
  (junction 7) -> (junction 10)
  data: ObjectsSortIndex function_input; ObjectsSortIndex_K1 function_input; StillTarget2_Dx function_input single size=1; StillTarget1_Dx function_input single size=1; StillTarget2_Dy function_input single size=1; StillTarget1_Dy function_input single size=1; StillTarget12_0_Theta function_output single size=1; RE_2TargetTheta_K1 function_input; C_TOS_StillObjSortInvalidIndex_Val parameter; RE_StationaryObjectsSortIndex input uint8 size=80; RE_StationaryObjectsSortIndex_K1 input; Object_Dx input single size=80; Object_Dy input single size=80; i local uint8 size=1 =1; StillTarget12_0_Theta local single size=1 =181; StillTarget23_12_Theta_ALL output single size=80 =ones(80,1)*181; StillTarget12_0_Theta_ALL output single size=80 =ones(80,1)*181; StillTarget23_12_Theta local single size=1 =181; C_TOS_RE_ThretaDefault_Val parameter; StillTarget1_Index local uint8 size=1 =0; StillTarget2_Index local uint8 size=1 =0; StillTarget2_Dx local single size=1 =255; StillTarget1_Dx local single size=1 =255; StillTarget1_Dy local single size=1 =255; StillTarget2_Dy local single size=1 =255; C_TOS_RE_80Single181Default_Val parameter; RE_2TargetTheta_ALL_K1 input; ObjectsSortIndex local uint8; ObjectsSortIndex_K1 local uint8; RE_2TargetTheta_K1 local single

== stateflow chart PubIfDecisionTOS_MDL/TOS_20201112/TOS_2012080320/PP1128/AAT-AdditionalAttributes/RoadEdge/RE_2020_12_07/RoadEdge_V2/TargetChain/EgoRightTargetChainDirection/TargetChainDirectionCalCulat ==
  note: RE_TargetChainDir
      | 0:Invalid
      | 1:Stright_Same  Dir
      | 2:Stright_Different Dir
      | 3:Left_Same  Dir
      | 4:Left_Different Dir
      | 5:Right_Same  Dir
      | 6:Right_Different Dir
  note: RE_TargetChainStartDir:
      |
      | 0:Invalid
      | 1:Stright Dir
      | 2:Left Dir
      | 3:Right Dir
  state TargetChainStartDirJudge [function]
    note: RE_TargetChainStartDir:
        |
        | 0:Invalid
        | 1:Stright  Dir
        | 2:Left Dir
        | 3:Right Dir
    (default) -> (junction 76)
    (junction 76) -> (junction 75) [order 1] : [RE_StillTarget_Theta2_ALL[i] < P_TOS_RE_StrightDirThetaMax_val &&...
        | RE_StillTarget_Theta2_ALL[i] > P_TOS_RE_StrightDirThetaMin_val]
    (junction 75) -> (junction 63) : {
        | RE_TargetChainStartDir[i] = uint8(1);
        | }
    (junction 76) -> (junction 68) [order 2]
    (junction 68) -> (junction 77) [order 1] : [RE_StillTarget_Theta2_ALL[i] <= P_TOS_RE_StrightDirThetaMin_val&&...
        | RE_StillTarget_Theta2_ALL[i] > single(-1)*C_TOS_RE_ThretaDefault_Val]
    (junction 68) -> (junction 64) [order 2]
    (junction 77) -> (junction 62) : {
        | RE_TargetChainStartDir[i]  = uint8(2);
        | }
    (junction 64) -> (junction 58) [order 1] : [RE_StillTarget_Theta2_ALL[i] >= P_TOS_RE_StrightDirThetaMax_val &&...
        | RE_StillTarget_Theta2_ALL[i] < C_TOS_RE_ThretaDefault_Val]
    (junction 64) -> (junction 59) [order 2] : {
        | RE_TargetChainStartDir[i]  = uint8(0);
        | }
        | %donothing
    (junction 58) -> (junction 61) : {
        | RE_TargetChainStartDir[i]  = uint8(3);
        | }
    (junction 63) -> (junction 62)
    (junction 61) -> (junction 59)
    (junction 62) -> (junction 61)
    (junction 59) -> (junction 80)
  state Target2ChainDirJudge [function]
    note: RE_TargetChainDir
        | 0:Invalid
        | 1:Stright_Same  Dir
        | 2:Stright_Different Dir
        | 3:Left_Same  Dir
        | 4:Left_Different Dir
        | 5:Right_Same  Dir
        | 6:Right_Different Dir
    state RightDir_TargetDirJudge [function]
      (default) -> (junction 282)
      (junction 282) -> (junction 285) [order 1] : [RE_StillTarget_Theta2_ALL[i] < P_TOS_RE_StrightDirThetaMax_val &&...
          | RE_StillTarget_Theta2_ALL[i] > P_TOS_RE_StrightDirThetaMin_val]
      (junction 282) -> (junction 300) [order 2]
      (junction 285) -> (junction 299) : {
          | RE_TargetChainDir[i] = uint8(5);
          | }
      (junction 300) -> (junction 286) [order 1] : [RE_StillTarget_Theta2_ALL[i] <= P_TOS_RE_StrightDirThetaMin_val &&...
          | RE_StillTarget_Theta2_ALL[i] > single(-1)*C_TOS_RE_ThretaDefault_Val]
      (junction 300) -> (junction 297) [order 2]
      (junction 286) -> (junction 289) : {
          | RE_TargetChainDir[i] = uint8(6);
          | }
      (junction 297) -> (junction 295) [order 1] : [RE_StillTarget_Theta2_ALL[i] >= P_TOS_RE_StrightDirThetaMax_val &&...
          | RE_StillTarget_Theta2_ALL[i]< C_TOS_RE_ThretaDefault_Val]
      (junction 297) -> (junction 278) [order 2] : {
          | RE_TargetChainDir[i] = uint8(0);
          | }%donothing
      (junction 295) -> (junction 292) : {
          | RE_TargetChainDir[i] = uint8(6);
          | }
      (junction 292) -> (junction 278)
      (junction 289) -> (junction 292)
      (junction 299) -> (junction 289)
      (junction 278) -> (junction 223)
    state LeftDir_TargetDirJudge [function]
      (default) -> (junction 256)
      (junction 256) -> (junction 258) [order 1] : [RE_StillTarget_Theta2_ALL[i] < P_TOS_RE_StrightDirThetaMax_val &&...
          | RE_StillTarget_Theta2_ALL[i] > P_TOS_RE_StrightDirThetaMin_val]
      (junction 256) -> (junction 265) [order 2]
      (junction 258) -> (junction 259) : {
          | RE_TargetChainDir[i] = uint8(3);
          | }
      (junction 265) -> (junction 267) [order 1] : [RE_StillTarget_Theta2_ALL[i] <= P_TOS_RE_StrightDirThetaMin_val &&...
          | RE_StillTarget_Theta2_ALL[i] > single(-1)*C_TOS_RE_ThretaDefault_Val]
      (junction 265) -> (junction 261) [order 2]
      (junction 267) -> (junction 273) : {
          | RE_TargetChainDir[i]  = uint8(4);
          | }
      (junction 261) -> (junction 270) [order 1] : [RE_StillTarget_Theta2_ALL[i] >= P_TOS_RE_StrightDirThetaMax_val &&...
          | RE_StillTarget_Theta2_ALL[i ]< C_TOS_RE_ThretaDefault_Val]
      (junction 261) -> (junction 254) [order 2] : {
          | RE_TargetChainDir[i] = uint8(0);
          | }%donothing
      (junction 270) -> (junction 268) : {
          | RE_TargetChainDir[i]  = uint8(4);
          | }
      (junction 259) -> (junction 273)
      (junction 273) -> (junction 268)
      (junction 268) -> (junction 254)
      (junction 254) -> (junction 276)
    state StrightDir_TargetDirJudge [function]
      (default) -> (junction 233)
      (junction 233) -> (junction 235) [order 1] : [RE_StillTarget_Theta2_ALL[i] < P_TOS_RE_StrightDirThetaMax_val &&...
          | RE_StillTarget_Theta2_ALL[i] > P_TOS_RE_StrightDirThetaMin_val]
      (junction 233) -> (junction 239) [order 2]
      (junction 235) -> (junction 230) : {
          | RE_TargetChainDir[i] = uint8(1);
          | }
      (junction 239) -> (junction 238) [order 1] : [RE_StillTarget_Theta2_ALL[i] <= P_TOS_RE_StrightDirThetaMin_val &&...
          | RE_StillTarget_Theta2_ALL[i] > single(-1)*C_TOS_RE_ThretaDefault_Val]
      (junction 239) -> (junction 243) [order 2]
      (junction 238) -> (junction 241) : {
          | RE_TargetChainDir[i] = uint8(2);
          | }
      (junction 243) -> (junction 227) [order 1] : [RE_StillTarget_Theta2_ALL[i] >= P_TOS_RE_StrightDirThetaMax_val &&...
          | RE_StillTarget_Theta2_ALL[i ]< C_TOS_RE_ThretaDefault_Val]
      (junction 243) -> (junction 229) [order 2] : {
          | RE_TargetChainDir[i] = uint8(0);
          | }%donothing
      (junction 227) -> (junction 246) : {
          | RE_TargetChainDir[i] = uint8(2);
          | }
      (junction 246) -> (junction 229)
      (junction 241) -> (junction 246)
      (junction 230) -> (junction 241)
      (junction 229) -> (junction 249)
    (default) -> (junction 114)
    (junction 114) -> (junction 113) [order 1] : [RE_TargetChainStartDir[i-uint8(1)] == uint8(1)]
    (junction 114) -> (junction 115) [order 2]
    (junction 113) -> (junction 250) : {
        | StrightDir_TargetDirJudge();
        | }
    (junction 115) -> (junction 116) [order 1] : [RE_TargetChainStartDir[i-uint8(1)]  == uint8(2)]
    (junction 115) -> (junction 117) [order 2]
    (junction 116) -> (junction 302) : {
        | LeftDir_TargetDirJudge();
        | }
    (junction 117) -> (junction 118) [order 1] : [RE_TargetChainStartDir[i-uint8(1)]  == uint8(3)]
    (junction 117) -> (junction 120) [order 2] : {
        | RE_TargetChainDir[i] = uint8(0);
        | }%donothing
    (junction 118) -> (junction 304) : {
        | RightDir_TargetDirJudge();
        | }
    (junction 304) -> (junction 120)
    (junction 302) -> (junction 304)
    (junction 250) -> (junction 302)
    (junction 120) -> (junction 123)
  (default) -> (junction 41)
  (junction 41) -> (junction 42) : {
      | i=uint8(1);
      | RE_TargetChainStartDir = C_TOS_RE_80Uint8Default_Val;
      | RE_TargetChainDir = C_TOS_RE_80Uint8Default_Val;
      |  }
      | %从第2个目标开始判断目标链起始方向
  (junction 42) -> (junction 47) [order 1] : [RE_StationaryObjectsSortIndex[i] ~= C_TOS_StillObjSortInvalidIndex_Val &&...
      | i <= uint8(79)]
  (junction 50) -> (junction 42) : {
      | i=i+uint8(1);
      | }
  (junction 42) -> (junction 44) [order 2]
  (junction 47) -> (junction 330) : {
      | TargetChainStartDirJudge();
      | }
  (junction 330) -> (junction 332) [order 1] : [i > uint8(1)]
      | %从第3个目标开始,判断目标链方向
  (junction 330) -> (junction 50) [order 2] : {
      | RE_TargetChainDir[i] = uint8(0);
      | }
  (junction 332) -> (junction 333) : {
      | Target2ChainDirJudge();
      | }
  (junction 333) -> (junction 50)
  (junction 44) -> (junction 45)
  data: RE_StationaryObjectsSortIndex input uint8 size=80; P_TOS_RE_StrightDirThetaMax_val parameter; C_TOS_RE_ThretaDefault_Val parameter; P_TOS_RE_StrightDirThetaMin_val parameter; RE_TargetChainStartDir output uint8 size=80; RE_TargetChainDir output uint8 size=80; i local uint8 size=1; RE_StillTarget_Theta2_ALL input single size=80; C_TOS_StillObjSortInvalidIndex_Val parameter; C_TOS_RE_80Uint8Default_Val parameter

== stateflow chart PubIfDecisionTOS_MDL/TOS_20201112/TOS_2012080320/PP1128/AAT-AdditionalAttributes/RoadEdge/RE_2020_12_07/RoadEdge_V2/TargetChain/EgoRightTargetChainDirection/Theta_Calculation ==
  state StillTarget12_0_Theta = Theta_Cal(ObjectsSortIndex,ObjectsSortIndex_K1,StillTarget2_Dx,StillTarget1_Dx,StillTarget2_Dy,StillTarget1_Dy,RE_2TargetTheta_K1) [function]
  (default) -> (junction 2) : {
      | i=uint8(1);
      | StillTarget12_0_Theta_ALL = C_TOS_RE_80Single181Default_Val;
      | StillTarget12_0_Theta_ALL[0] = single(90);
      | StillTarget23_12_Theta_ALL = C_TOS_RE_80Single181Default_Val;
      | }
      | %从第2个目标开始   1
  (junction 2) -> (junction 3) [order 1] : [RE_StationaryObjectsSortIndex[i] ~= C_TOS_StillObjSortInvalidIndex_Val &&...
      | i <= uint8(79)]
  (junction 76) -> (junction 2) : {
      | i = i+uint8(1);
      | }
  (junction 2) -> (junction 7) [order 2]
  (junction 3) -> (junction 33) : {
      | StillTarget1_Index=RE_StationaryObjectsSortIndex[i-uint8(1)];
      | StillTarget2_Index=RE_StationaryObjectsSortIndex[i];
      | }
  (junction 33) -> (junction 12) : {
      | StillTarget1_Dx = Object_Dx[StillTarget1_Index-uint8(1)];
      | StillTarget2_Dx = Object_Dx[StillTarget2_Index-uint8(1)];
      | StillTarget1_Dy = Object_Dy[StillTarget1_Index-uint8(1)];
      | StillTarget2_Dy = Object_Dy[StillTarget2_Index-uint8(1)];
      | }
      | %提取相邻两个点的Dx，Dy
  (junction 12) -> (junction 74) : {
      | ObjectsSortIndex_K1 = RE_StationaryObjectsSortIndex_K1[i];
      | ObjectsSortIndex = RE_StationaryObjectsSortIndex[i];
      | RE_2TargetTheta_K1 = RE_2TargetTheta_ALL_K1[i];
      | StillTarget12_0_Theta = Theta_Cal(ObjectsSortIndex,ObjectsSortIndex_K1,StillTarget2_Dx,StillTarget1_Dx,StillTarget2_Dy,StillTarget1_Dy,RE_2TargetTheta_K1);
      | StillTarget12_0_Theta_ALL[i] = StillTarget12_0_Theta;
      | }
      | %计算相邻两个点的直线与dy轴夹角，角度范围，顺时针0-180度
  (junction 74) -> (junction 76) : {
      | StillTarget23_12_Theta = StillTarget12_0_Theta_ALL[i] - StillTarget12_0_Theta_ALL[i-uint8(1)];
      | StillTarget23_12_Theta_ALL[i] = StillTarget23_12_Theta;
      | }
      | %计算2，3点连线的斜率角减去第1，2点连线之间的斜率角，角度范围+-180度
      | %StillTarget23_12_Theta_ALL元素对应按Dx从小到大的顺序排列
  (junction 7) -> (junction 10)
  data: ObjectsSortIndex function_input; ObjectsSortIndex_K1 function_input; StillTarget2_Dx function_input single size=1; StillTarget1_Dx function_input single size=1; StillTarget2_Dy function_input single size=1; StillTarget1_Dy function_input single size=1; StillTarget12_0_Theta function_output single size=1; RE_2TargetTheta_K1 function_input; C_TOS_StillObjSortInvalidIndex_Val parameter; RE_StationaryObjectsSortIndex input uint8 size=80; RE_StationaryObjectsSortIndex_K1 input; Object_Dx input single size=80; Object_Dy input single size=80; i local uint8 size=1 =1; StillTarget12_0_Theta local single size=1 =181; StillTarget23_12_Theta_ALL output single size=80 =ones(80,1)*181; StillTarget12_0_Theta_ALL output single size=80 =ones(80,1)*181; StillTarget23_12_Theta local single size=1 =181; C_TOS_RE_ThretaDefault_Val parameter; StillTarget1_Index local uint8 size=1 =0; StillTarget2_Index local uint8 size=1 =0; StillTarget2_Dx local single size=1 =255; StillTarget1_Dx local single size=1 =255; StillTarget1_Dy local single size=1 =255; StillTarget2_Dy local single size=1 =255; C_TOS_RE_80Single181Default_Val parameter; RE_2TargetTheta_ALL_K1 input; ObjectsSortIndex local uint8; ObjectsSortIndex_K1 local uint8; RE_2TargetTheta_K1 local single
